simulink model "Suspen_mode"  (R2023a)
settings: Solver=VariableStepAuto  StartTime=0.0  StopTime=15  RelTol=1e-3
values from neighbouring files (symbols this model uses):
  b1 = 1000    [suspencion.m]
  k1 = 16182    [suspencion.m]
  k2 = 19000    [suspencion.m]
  m1 = 290    [suspencion.m]
  m2 = 59    [suspencion.m]

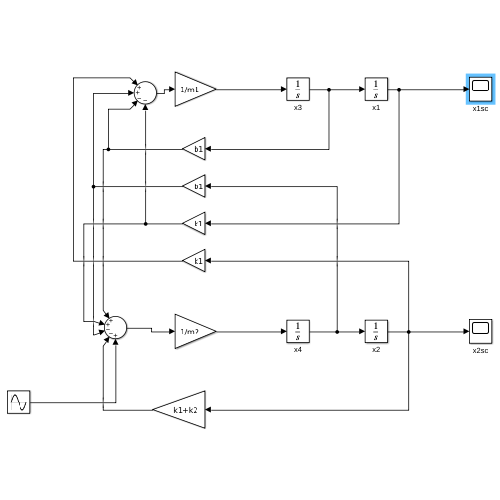
[thumbnail: Simulink's stored preview of the top-level diagram]
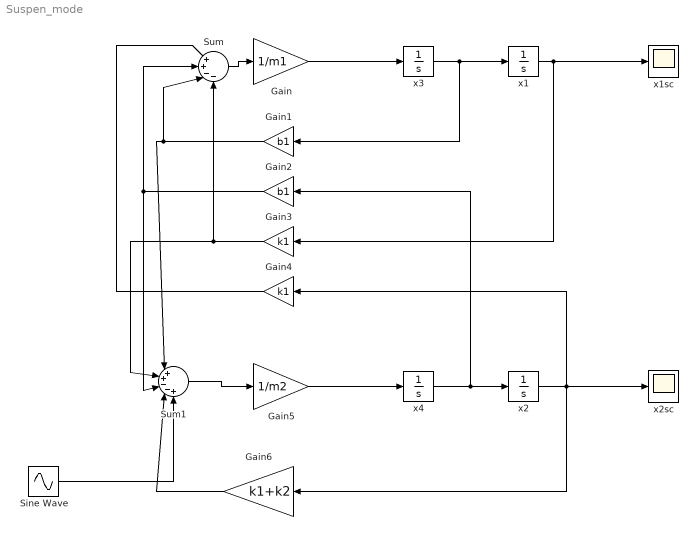
== system Suspen_mode ==
  Gain : Gain  Gain=1/m1
  Gain1 : Gain  Gain=b1
  Gain2 : Gain  Gain=b1
  Gain3 : Gain  Gain=k1
  Gain4 : Gain  Gain=k1
  Gain5 : Gain  Gain=1/m2
  Gain6 : Gain  Gain=k1+k2
  Sine Wave : Sin  Amplitude=0.05*k2  Frequency=pi*0.5  SampleTime=0
  Sum : Sum  Inputs=|++--
  Sum1 : Sum  Inputs=|++--+
  x{1..4} (4 alike) : Integrator
  x1sc : Scope
  x2sc : Scope
  wires:
  x3/1 -> Gain1/1, x1/1
  x4/1 -> Gain2/1, x2/1
  Sum/1 -> Gain/1
  Gain/1 -> x3/1
  Gain1/1 -> Sum1/1, Sum/3
  Gain2/1 -> Sum1/3, Sum/2
  x1/1 -> Gain3/1, x1sc/1
  x2/1 -> Gain6/1, Gain4/1, x2sc/1
  Gain3/1 -> Sum1/2, Sum/4
  Gain4/1 -> Sum/1
  Gain5/1 -> x4/1
  Sum1/1 -> Gain5/1
  Gain6/1 -> Sum1/4
  Sine Wave/1 -> Sum1/5
